simulink library "synaptic_scaling_choice"  (R2013a)
settings: Solver=ode45  StartTime=0.0  StopTime=10.0  RelTol=1e-3
undefined symbols (not defined in the file): lambda1, lambda3, lambda4, w_0
libraries: WaveformsLib x1, synaptic_scaling_choice x1
settings Model: Creator=Leo  LastModifiedBy=Leo

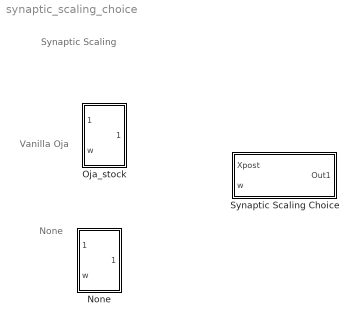
== system synaptic_scaling_choice ==
  note: None
  note: Vanilla Oja
  note: Synaptic Scaling
  None : Subsystem
  Oja_stock : Subsystem
  Synaptic Scaling Choice : Subsystem  BlockChoice=Oja_stock
      settings: TemplateBlock=self  MemberBlocks=None,Oja_stock

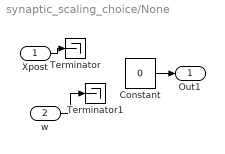
== system synaptic_scaling_choice/None ==
  Xpost : Inport
  w : Inport  Port=2
  Constant : Constant  Value=0
  Terminator : Terminator
  Terminator1 : Terminator
  Out1 : Outport
  wires:
  Constant/1 -> Out1/1
  w/1 -> Terminator1/1
  Xpost/1 -> Terminator/1

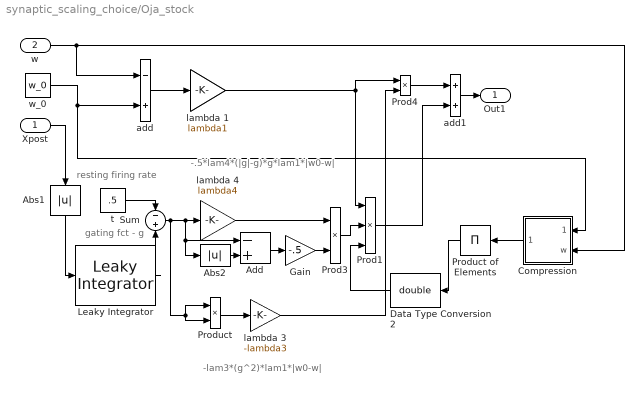
== system synaptic_scaling_choice/Oja_stock ==
  note: resting firing rate
  note: -lam3*(g^2)*lam1*|w0-w|
  note: -.5*lam4*(|g|-g)*g*lam1*|w0-w|
  note: gating fct - g
  Xpost : Inport
  w : Inport  Port=2
  Abs1 : Abs
  Abs2 : Abs
  Add : Sum  Inputs=-+
  Compression : Subsystem
  Data Type Conversion2 : DataTypeConversion  OutDataTypeStr=double
  Gain : Gain  Gain=-.5
  Leaky Integrator : WaveformsLib/Leaky Integrator  X0=0  A=0.01
  Prod1 : Product  Inputs=3  RndMeth=Zero
  Prod3 : Product  RndMeth=Zero
  Prod4 : Product  RndMeth=Zero
  Product : Product  RndMeth=Zero
  Product of Elements : Product  Inputs=*  OutDataTypeStr=double
  Sum : Sum  Inputs=-+
  add : Sum  Inputs=-+
  add1 : Sum
  lambda 1 : Gain  Gain=lambda1
  lambda 3 : Gain  Gain=-lambda3
  lambda 4 : Gain  Gain=lambda4
  t : Constant  Value=.5
  w_0 : Constant  Value=w_0
  Out1 : Outport
  wires:
  w_0/1 -> add/2, Compression/1(w_0)
  Xpost/1 -> Abs1/1
  lambda 1/1 -> Prod4/1, Prod1/1
  t/1 -> Sum/1
  Sum/1 -> lambda 4/1, Add/1, Abs2/1, Product/1, Product/2
  Leaky Integrator/1 -> Sum/2
  Abs1/1 -> Leaky Integrator/1
  Abs2/1 -> Add/2
  Add/1 -> Gain/1
  Gain/1 -> Prod3/2
  Prod3/1 -> Prod1/2
  lambda 3/1 -> Prod4/2
  Prod1/1 -> add1/2
  Product/1 -> lambda 3/1
  lambda 4/1 -> Prod3/1
  Compression/1(Out1) -> Product of Elements/1
  Product of Elements/1 -> Data Type Conversion2/1
  w/1 -> add/1, Compression/2(w)
  Data Type Conversion2/1 -> Prod1/3
  add/1 -> lambda 1/1
  Prod4/1 -> add1/1
  add1/1 -> Out1/1

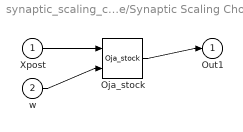
== system synaptic_scaling_choice/Synaptic Scaling Choice ==
  Xpost : Inport
  w : Inport  Port=2
  Oja_stock : synaptic_scaling_choice/Oja_stock
  Out1 : Outport
  wires:
  Xpost/1 -> Oja_stock/1
  w/1 -> Oja_stock/2
  Oja_stock/1 -> Out1/1

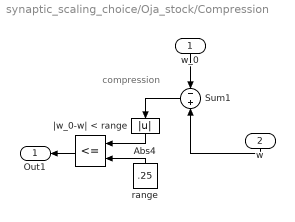
== system synaptic_scaling_choice/Oja_stock/Compression ==
  note: compression
  w_0 : Inport
  w : Inport  Port=2
  Abs4 : Abs
  Sum1 : Sum  Inputs=-+
  range : Constant  Value=.25
  |w_0-w| < range : RelationalOperator  Operator=<=  OutDataTypeStr=boolean
  Out1 : Outport
  wires:
  Sum1/1 -> Abs4/1
  range/1 -> |w_0-w| < range/2
  Abs4/1 -> |w_0-w| < range/1
  w_0/1 -> Sum1/1
  w/1 -> Sum1/2
  |w_0-w| < range/1 -> Out1/1
